simulink model "Filter_attivo"  (R2016b)
settings: Solver=ode23t  StartTime=0.0  StopTime=2.4  MaxStep=1e-4  RelTol=1e-3  EnableMultiTasking=on
values from neighbouring files (symbols this model uses):
  ampiezza_rete = 150/sqrt(3)    [Data.m]    (also in taratura.m)
  C = 2.2e-3    (= 0.0022)    [Data.m]
  C_raddr = 600e-6    (= 0.0006)    [Data.m]
  f = 50    [Data.m]    (also in Spettro_complesso.m = bar(-fp((26:25:25000-25)),PyTHD(length(PyTHD)-1:-1:length(Py)
  f_am = 500    [Data.m]
  h = Lagrange_coef(f,1/Tc)    [Data.m]    (also in Lagrange_coef.m = NaN(4,round(fc/f1*0.5)))
  h_rit = Lagrange_coef_rit(1.5)    [Data.m]
  k_interno = 0.99    [tuning.m]
  k_par_AM = 10    [Data.m]
  ki_PI = 0.2    [Data.m]
  ki_PLL = 1000    [Data.m]
  ki_ris = 47.5*2    (= 95)    [Data.m]
  kp_PI = 1.57    [Data.m]
  kp_PLL = 0.9    [Data.m]
  kp_ris = 47.5*0.089*2    (= 8.455)    [Data.m]
  L_disaccoppiamento = 2*1.18e-3    (= 0.00236)    [Data.m]    (also in taratura.m)
  L_rete = 4e-3    (= 0.004)    [Data.m]    (also in tuning.m)
  max_PI = 8    [Data.m]
  max_PLL = 1000    [Data.m]
  min_PI = -8    [Data.m]
  min_PLL = -1000    [Data.m]
  Notch_z = 1-Peaking_z    [Data.m]
  Notch_z_AM1 = 1-Peaking_z_AM1    [Notch.m]
  peak_rete = Peaking(f,1/Tc,0.1)    [Data.m]
  Peaking_dir1_d = c2d(Peaking_dir1_s,1/fs,'tustin')    [semipeaking.m]
  pendenza = 1000    [Data.m]
  R_carico = 50    [Data.m]
  R_disaccoppiamento = 2*13e-3    (= 0.026)    [Data.m]    (also in taratura.m)
  R_raddr = 60    [Data.m]
  R_rete = 100e-3    (= 0.1)    [Data.m]    (also in tuning.m = 0.01)
  T = 20e-3    (= 0.02)    [Data.m]    (also in tuning.m)
  tau_filtro_Vdc_ref = 0.15    [Data.m]
  Tc = 1/10000    (= 0.0001)    [Data.m]    (also in taratura.m; tuning.m)
  Vdc_ref = 200    [Data.m]    (also in taratura.m)
  w_filtro = 2*pi*f_taglio    (= 56548.6677646)    [Data.m]
undefined symbols (not defined in the file or in its folder): DiscIntNeverNeededParam, k_par, k_ser, Notch_z_AM1_5, Notch_z_AM1_7, Notch_z_AM2_5, Notch_z_AM2_7, Peaking_inv_d, plecs, Q_inv
libraries: powerlib x54, simulink x8, powerlib_extras x4, powerlib_meascontrol x2
(part 1 of 5)
settings Model: SimulationMode=accelerator  Creator=utente  LastModifiedBy=franc
settings DataIOCC: SaveFormat=Array
settings OptimizationCC: ExpressionDepthLimit=2147483647  EfficientMapNaN2IntZero=off  LifeSpan=inf
settings DebuggingCC: UnderspecifiedInitializationDetection=Classic  MergeDetectMultiDrivingBlocksExec=none  MaxConsecutiveZCsMsg=none  SolverPrmCheckMsg=warning  FcnCallInpInsideContextMsg=warning  AllowSymbolicDim=off  StateNameClashWarn=warning  SFUnexpectedBacktrackingDiag=warning  SFNoUnconditionalDefaultTransitionDiag=warning  SFExecutionAtInitializationDiag=none
settings HardwareCC: ProdBitPerPointer=32  ProdBitPerSizeT=32  ProdBitPerPtrDiffT=32  ProdLargestAtomicFloat=None  ProdIntDivRoundTo=Undefined  ProdEndianess=Unspecified  ProdWordSize=32  ProdHWDeviceType=32-bit Generic  TargetBitPerPointer=64  TargetBitPerSizeT=64  TargetBitPerPtrDiffT=64  TargetLongLongMode=on  TargetIntDivRoundTo=Zero  TargetEndianess=LittleEndian  TargetWordSize=64  TargetHWDeviceType=MATLAB Host  ProdEqTarget=off
settings ModelReferenceCC: PropagateSignalLabelsOutOfModel=off
settings SFSimCC: SimParseCustomCode=off
settings CodeAppCC: MaxIdLength=128
settings GRTTargetCC: TargetLangStandard=C89/C90 (ANSI)  CombineOutputUpdateFcns=off  GRTInterface=on
settings ConfigComp: CovMetricSettings=dw  CovHtmlReporting=on  CovSaveCumulativeToWorkspaceVar=on  CovSaveSingleToWorkspaceVar=on  CovExternalEMLEnable=off  CovSFcnEnable=off

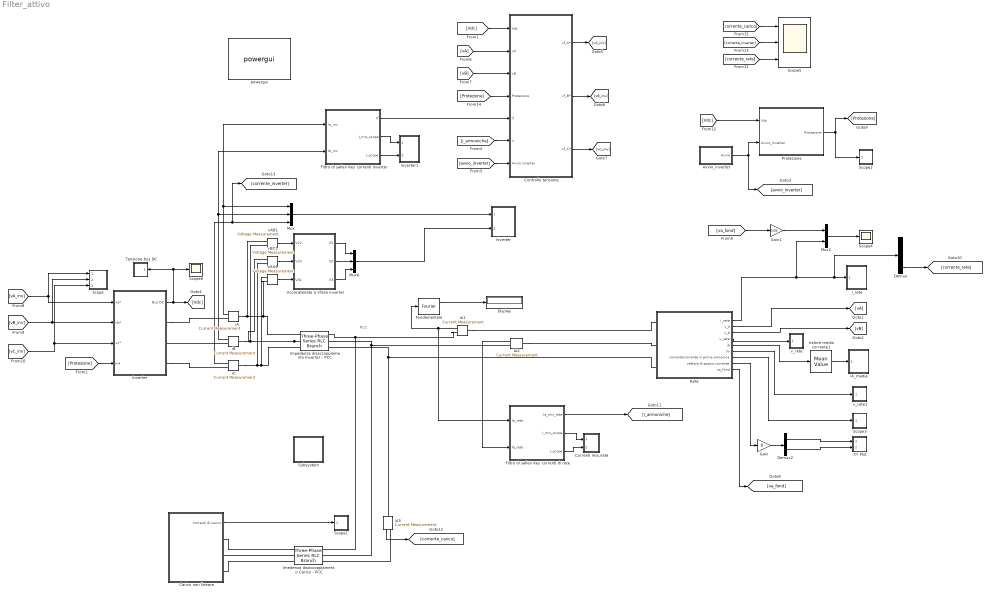
== system Filter_attivo ==
  note: PCC
  Avvio_inverter : Subsystem  mask{avvio=0.2}
      mask prompts: avvio "Istante avvio inverter"
  Carico non lineare : Subsystem
  Controllo tensione : Subsystem
  Correnti misurate : Subsystem  LoadFcn=plecs('sl', 300);  InitFcn=plecs('sl', 314);  StartFcn=plecs('sl', 308);  StopFcn=plecs('sl', 309);  mask{Settings=<binary blob, 300 chars, not shown>}
      mask init:
      | plecs('sl', 315);
      settings: CopyFcn=plecs('sl', 303);  DeleteFcn=plecs('sl', 305);  UndoDeleteFcn=plecs('sl', 306);  PreSaveFcn=plecs('sl', 311);  NameChangeFcn=plecs('sl', 310);  DestroyFcn=plecs('sl', 307);  OpenFcn=plecs('sl', 302);  ErrorFcn=plerrorfcn
      mask Display: plot([0.1 0.9 0.9 0.1 0.1], [0.9 0.9 0.5 0.5 0.9])
  Demux : Demux  Outputs=3
  Demux2 : Demux  Outputs=2
  Display : Display
  "Filtro di sallen Key correnti inverter " : Subsystem
  Filtro di sallen Key correnti di rete : Subsystem
  Fondamentale : powerlib_meascontrol/Measurements/Fourier  Freq=50  n=1  InInit=[0, 0]  Ts=0
  Gain : Gain  Gain=0
  Gain1 : Gain  Gain=0.05
  Imedenza disaccoppiamento Carico - PCC : powerlib/Elements/Three-Phase Series RLC Branch  LConnTagsString=A|B|C  RConnTagsString=A|B|C  BranchType=RL  Resistance=R_disaccoppiamento  Inductance=L_disaccoppiamento  Capacitance=1e-6  Measurements=None
  Impedenza disaccoppiamento Inverter - PCC : powerlib/Elements/Three-Phase Series RLC Branch  LConnTagsString=A|B|C  RConnTagsString=A|B|C  BranchType=RL  Resistance=R_disaccoppiamento  Inductance=L_disaccoppiamento  Capacitance=1e-6  Measurements=None
  Inverter : Subsystem  LoadFcn=plecs('sl', 300);  InitFcn=plecs('sl', 314);  StartFcn=plecs('sl', 308);  StopFcn=plecs('sl', 309);  mask{Settings=<binary blob, 1152 chars, not shown>}
      mask init:
      | plecs('sl', 315);
      settings: CopyFcn=plecs('sl', 303);  DeleteFcn=plecs('sl', 305);  UndoDeleteFcn=plecs('sl', 306);  PreSaveFcn=plecs('sl', 311);  NameChangeFcn=plecs('sl', 310);  DestroyFcn=plecs('sl', 307);  OpenFcn=plecs('sl', 302);  ErrorFcn=plerrorfcn
      mask Display: plot([0.1 0.9 0.9 0.1 0.1], [0.9 0.9 0.5 0.5 0.9])
  "Inverter " : Subsystem
  Inverter1 : Subsystem  LoadFcn=plecs('sl', 300);  InitFcn=plecs('sl', 314);  StartFcn=plecs('sl', 308);  StopFcn=plecs('sl', 309);  mask{Settings=<binary blob, 1020 chars, not shown>}
      mask init:
      | plecs('sl', 315);
      settings: CopyFcn=plecs('sl', 303);  DeleteFcn=plecs('sl', 305);  UndoDeleteFcn=plecs('sl', 306);  PreSaveFcn=plecs('sl', 311);  NameChangeFcn=plecs('sl', 310);  DestroyFcn=plecs('sl', 307);  OpenFcn=plecs('sl', 302);  ErrorFcn=plerrorfcn
      mask Display: plot([0.1 0.9 0.9 0.1 0.1], [0.9 0.9 0.5 0.5 0.9])
  Mux : Mux  Inputs=3
  Mux2 : Mux  Inputs=2
  Mux6 : Mux  Inputs=3
  Protezione : Subsystem  mask{limite_up=250, limite_down=70}
      mask prompts: limite_up "tensione max bus DC"; limite_down "tensione min bus DC"
  Rete : Subsystem
  Scope : Subsystem  LoadFcn=plecs('sl', 300);  InitFcn=plecs('sl', 314);  StartFcn=plecs('sl', 308);  StopFcn=plecs('sl', 309);  mask{Settings=<binary blob, 1148 chars, not shown>}
      mask init:
      | plecs('sl', 315);
      settings: CopyFcn=plecs('sl', 303);  DeleteFcn=plecs('sl', 305);  UndoDeleteFcn=plecs('sl', 306);  PreSaveFcn=plecs('sl', 311);  NameChangeFcn=plecs('sl', 310);  DestroyFcn=plecs('sl', 307);  OpenFcn=plecs('sl', 302);  ErrorFcn=plerrorfcn
      mask Display: plot([0.1 0.9 0.9 0.1 0.1], [0.9 0.9 0.5 0.5 0.9])
  Scope1 : Subsystem  LoadFcn=plecs('sl', 300);  InitFcn=plecs('sl', 314);  StartFcn=plecs('sl', 308);  StopFcn=plecs('sl', 309);  mask{Settings=<binary blob, 876 chars, not shown>}
      mask init:
      | plecs('sl', 315);
      settings: CopyFcn=plecs('sl', 303);  DeleteFcn=plecs('sl', 305);  UndoDeleteFcn=plecs('sl', 306);  PreSaveFcn=plecs('sl', 311);  NameChangeFcn=plecs('sl', 310);  DestroyFcn=plecs('sl', 307);  OpenFcn=plecs('sl', 302);  ErrorFcn=plerrorfcn
      mask Display: plot([0.1 0.9 0.9 0.1 0.1], [0.9 0.9 0.5 0.5 0.9])
  Scope2 : Subsystem  LoadFcn=plecs('sl', 300);  InitFcn=plecs('sl', 314);  StartFcn=plecs('sl', 308);  StopFcn=plecs('sl', 309);  mask{Settings=<binary blob, 892 chars, not shown>}
      mask init:
      | plecs('sl', 315);
      settings: CopyFcn=plecs('sl', 303);  DeleteFcn=plecs('sl', 305);  UndoDeleteFcn=plecs('sl', 306);  PreSaveFcn=plecs('sl', 311);  NameChangeFcn=plecs('sl', 310);  DestroyFcn=plecs('sl', 307);  OpenFcn=plecs('sl', 302);  ErrorFcn=plerrorfcn
      mask Display: plot([0.1 0.9 0.9 0.1 0.1], [0.9 0.9 0.5 0.5 0.9])
  Scope3 : Subsystem  LoadFcn=plecs('sl', 300);  InitFcn=plecs('sl', 314);  StartFcn=plecs('sl', 308);  StopFcn=plecs('sl', 309);  mask{Settings=<binary blob, 892 chars, not shown>}
      mask init:
      | plecs('sl', 315);
      settings: CopyFcn=plecs('sl', 303);  DeleteFcn=plecs('sl', 305);  UndoDeleteFcn=plecs('sl', 306);  PreSaveFcn=plecs('sl', 311);  NameChangeFcn=plecs('sl', 310);  DestroyFcn=plecs('sl', 307);  OpenFcn=plecs('sl', 302);  ErrorFcn=plerrorfcn
      mask Display: plot([0.1 0.9 0.9 0.1 0.1], [0.9 0.9 0.5 0.5 0.9])
  Scope4 : Scope
  Scope5 : Scope  NumInputPorts=3
  Scope6 : Scope
  Subsystem : Subsystem
  Tensione bus DC : Subsystem  LoadFcn=plecs('sl', 300);  InitFcn=plecs('sl', 314);  StartFcn=plecs('sl', 308);  StopFcn=plecs('sl', 309);  mask{Settings=<binary blob, 960 chars, not shown>}
      mask init:
      | plecs('sl', 315);
      settings: CopyFcn=plecs('sl', 303);  DeleteFcn=plecs('sl', 305);  UndoDeleteFcn=plecs('sl', 306);  PreSaveFcn=plecs('sl', 311);  NameChangeFcn=plecs('sl', 310);  DestroyFcn=plecs('sl', 307);  OpenFcn=plecs('sl', 302);  ErrorFcn=plerrorfcn
      mask Display: plot([0.1 0.9 0.9 0.1 0.1], [0.9 0.9 0.5 0.5 0.9])
  Valore medio corrente1 : powerlib_extras/Measurements/Mean Value  Period=3*Tc
  Vconcatenate a Vfase inverter : Subsystem
  XY Plot : Subsystem  LoadFcn=plecs('sl', 317);  InitFcn=plecs('sl', 314);  StartFcn=plecs('sl', 308);  StopFcn=plecs('sl', 309);  mask{Settings=<binary blob, 592 chars, not shown>}
      mask init:
      | plecs('sl', 315);
      settings: CopyFcn=plecs('sl', 318);  DeleteFcn=plecs('sl', 305);  UndoDeleteFcn=plecs('sl', 306);  PreSaveFcn=plecs('sl', 311);  NameChangeFcn=plecs('sl', 310);  DestroyFcn=plecs('sl', 307);  OpenFcn=plecs('sl', 302);  ErrorFcn=plerrorfcn
      mask Display:
      | plot([0.05 0.95 0.95 0.05 0.05], [0.95 0.95 0.05 0.05 0.95])
      | plot(0.5+sin((0:0.2:2)*pi)*0.3, 0.5+sin((0:0.2:2)*pi + pi/4)*0.3);
  iA{,1..2,5} (4 alike) : powerlib/Measurements/Current Measurement  PhasorSimulation=off  OutputType=Complex  PSBequivalent=0
  iA_media : Subsystem  LoadFcn=plecs('sl', 300);  InitFcn=plecs('sl', 314);  StartFcn=plecs('sl', 308);  StopFcn=plecs('sl', 309);  mask{Settings=<binary blob, 892 chars, not shown>}
      mask init:
      | plecs('sl', 315);
      settings: CopyFcn=plecs('sl', 303);  DeleteFcn=plecs('sl', 305);  UndoDeleteFcn=plecs('sl', 306);  PreSaveFcn=plecs('sl', 311);  NameChangeFcn=plecs('sl', 310);  DestroyFcn=plecs('sl', 307);  OpenFcn=plecs('sl', 302);  ErrorFcn=plerrorfcn
      mask Display: plot([0.1 0.9 0.9 0.1 0.1], [0.9 0.9 0.5 0.5 0.9])
  iB : powerlib/Measurements/Current Measurement  PhasorSimulation=off  OutputType=Complex  PSBequivalent=0
  iC : powerlib/Measurements/Current Measurement  PhasorSimulation=off  OutputType=Complex  PSBequivalent=0
  i_rete : Subsystem  LoadFcn=plecs('sl', 300);  InitFcn=plecs('sl', 314);  StartFcn=plecs('sl', 308);  StopFcn=plecs('sl', 309);  mask{Settings=<binary blob, 1020 chars, not shown>}
      mask init:
      | plecs('sl', 315);
      settings: CopyFcn=plecs('sl', 303);  DeleteFcn=plecs('sl', 305);  UndoDeleteFcn=plecs('sl', 306);  PreSaveFcn=plecs('sl', 311);  NameChangeFcn=plecs('sl', 310);  DestroyFcn=plecs('sl', 307);  OpenFcn=plecs('sl', 302);  ErrorFcn=plerrorfcn
      mask Display: plot([0.1 0.9 0.9 0.1 0.1], [0.9 0.9 0.5 0.5 0.9])
  powergui : powerlib/powergui  SimulationMode=Continuous  SolverType=Tustin  SampleTime=50e-6  frequency=60  SPID=off  DisableSnubberDevices=off  DisableRonSwitches=off  DisableVfSwitches=off  SwTol=0  DisplayEquations=off  Interpol=off  ExternalGateDelay=off  methode=off  Ts=0  FunctionMessages=off  echomessages=off  HookPort=off  EnableUseOfTLC=off  x0status=blocks  frequencyindice=0  Pbase=100e6  ErrMax=1e-4  Iterations=50  UnitsV=kV  UnitsW=MW  buscounter=0  RestoreLinks=warning  ResistiveCurrentMeasurement=off  Frange=[0:2:500]  Ylog=off  Xlog=on  ShowGrid=off  save=off  variable=ZData  structure=logsout  ZoomFFT=off  StartTime=1  cycles=5  DisplayStyle=1  fundamental=50  FreqAxis=off  MaxFrequency=10000  frequencyindicesteady=1  RmsSteady=1  display=off
  vAB1 : powerlib/Measurements/Voltage Measurement  PhasorSimulation=off  OutputType=Complex  PSBequivalent=0
  vBC1 : powerlib/Measurements/Voltage Measurement  PhasorSimulation=off  OutputType=Complex  PSBequivalent=0
  vCA1 : powerlib/Measurements/Voltage Measurement  PhasorSimulation=off  OutputType=Complex  PSBequivalent=0
  v_rete : Subsystem  LoadFcn=plecs('sl', 300);  InitFcn=plecs('sl', 314);  StartFcn=plecs('sl', 308);  StopFcn=plecs('sl', 309);  mask{Settings=<binary blob, 892 chars, not shown>}
      mask init:
      | plecs('sl', 315);
      settings: CopyFcn=plecs('sl', 303);  DeleteFcn=plecs('sl', 305);  UndoDeleteFcn=plecs('sl', 306);  PreSaveFcn=plecs('sl', 311);  NameChangeFcn=plecs('sl', 310);  DestroyFcn=plecs('sl', 307);  OpenFcn=plecs('sl', 302);  ErrorFcn=plerrorfcn
      mask Display: plot([0.1 0.9 0.9 0.1 0.1], [0.9 0.9 0.5 0.5 0.9])
  v_rete1 : Subsystem  LoadFcn=plecs('sl', 300);  InitFcn=plecs('sl', 314);  StartFcn=plecs('sl', 308);  StopFcn=plecs('sl', 309);  mask{Settings=<binary blob, 892 chars, not shown>}
      mask init:
      | plecs('sl', 315);
      settings: CopyFcn=plecs('sl', 303);  DeleteFcn=plecs('sl', 305);  UndoDeleteFcn=plecs('sl', 306);  PreSaveFcn=plecs('sl', 311);  NameChangeFcn=plecs('sl', 310);  DestroyFcn=plecs('sl', 307);  OpenFcn=plecs('sl', 302);  ErrorFcn=plerrorfcn
      mask Display: plot([0.1 0.9 0.9 0.1 0.1], [0.9 0.9 0.5 0.5 0.9])
  wires:
  [Vdc] -> Controllo tensione/1(Vdc)
  iB/1 -> "Filtro di sallen Key correnti inverter "/2(Ib_inv), Mux/2
  iA/1 -> "Filtro di sallen Key correnti inverter "/1(Ia_inv), Mux/1
  [vA] -> Controllo tensione/2(vA)
  [vB] -> Controllo tensione/3(vB)
  iC/1 -> [corrente_inverter], Mux/3
  Controllo tensione/3(vf_C*) -> [vC_inv]
  Controllo tensione/2(vf_B*) -> [vB_inv]
  Controllo tensione/1(vf_A*) -> [vA_inv]
  [Protezione] -> Controllo tensione/4(Protezione)
  vAB1/1 -> Vconcatenate a Vfase inverter/1(V12)
  vBC1/1 -> Vconcatenate a Vfase inverter/2(V23)
  vCA1/1 -> Vconcatenate a Vfase inverter/3(V31)
  Vconcatenate a Vfase inverter/2(E2) -> Mux6/2
  Vconcatenate a Vfase inverter/1(E1) -> Mux6/1
  Vconcatenate a Vfase inverter/3(E3) -> Mux6/3
  "Filtro di sallen Key correnti inverter "/2(I_mis_scope) -> Inverter1/1(1)
  "Filtro di sallen Key correnti inverter "/3(I_scope) -> Inverter1/2(2)
  "Filtro di sallen Key correnti inverter "/1(If) -> Controllo tensione/5(if)
  Protezione/1("Protezione ") -> Scope2/1(1), [Protezione]
  [Vdc] -> Protezione/1(Vdc)
  [vA_inv] -> Scope/1(1), "Inverter "/1(va*)
  [vB_inv] -> Scope/2(2), "Inverter "/2(vb*)
  [vC_inv] -> Scope/3(3), "Inverter "/3(vc*)
  [Protezione] -> "Inverter "/4(In4)
  "Inverter "/1(Bus DC) -> Scope6/1, Tensione bus DC/1(1), [Vdc]
  Rete/2(v_a) -> [vA]
  Rete/3(v_b) -> [vB]
  [i_armoniche] -> Controllo tensione/6(ir)
  iA1/1 -> Filtro di sallen Key correnti di rete/1(Ia_rete), Fondamentale/1
  Carico non lineare/1(Correnti di carico) -> Scope1/1(1)
  Fondamentale/1 -> Display/1
  iA2/1 -> Filtro di sallen Key correnti di rete/2(Ib_rete)
  Filtro di sallen Key correnti di rete/2(I_mis_scope) -> Correnti misurate/1(1)
  Filtro di sallen Key correnti di rete/3(I_scope) -> Correnti misurate/2(2)
  Filtro di sallen Key correnti di rete/1(Ia_mis_rete) -> [i_armoniche]
  Rete/4("v_rete ") -> v_rete/1(1)
  iA5/1 -> [corrente_carico]
  Rete/1("i_rete ") -> Mux2/2, Demux/1, i_rete/1(1)
  Avvio_inverter/1(Avvio) -> [avvio_inverter], Protezione/2(Avvio_inverter)
  Mux/1 -> Inverter/1(1)
  Mux6/1 -> Inverter/2(2)
  Rete/5(iA) -> Valore medio corrente1/1
  Valore medio corrente1/1 -> iA_media/1(1)
  [avvio_inverter] -> Controllo tensione/7("Avvio inverter ")
  Rete/6(i/v) -> v_rete1/1(1)
  Rete/7(corrente/corrente in prima armonica) -> Scope3/1(1)
  Rete/8(vettore di spazio corrente) -> Gain/1
  Demux2/1 -> XY Plot/1(1)
  Demux2/2 -> XY Plot/2(2)
  Gain/1 -> Demux2/1
  Mux2/1 -> Scope4/1
  Gain1/1 -> Mux2/1
  [va_fond] -> Gain1/1
  Rete/9(va_fond) -> [va_fond]
  Demux/3 -> [corrente_rete]
  [corrente_rete] -> Scope5/3
  [corrente_inverter] -> Scope5/2
  [corrente_carico] -> Scope5/1
  connections:
  vAB1/LConn1 -- iA/LConn1 -- vCA1/LConn2 -- Impedenza disaccoppiamento Inverter - PCC/LConn1
  Impedenza disaccoppiamento Inverter - PCC/LConn2 -- iB/LConn1 -- vBC1/LConn1 -- vAB1/LConn2
  vBC1/LConn2 -- vCA1/LConn1 -- Impedenza disaccoppiamento Inverter - PCC/LConn3 -- iC/LConn1
  Imedenza disaccoppiamento Carico - PCC/LConn2 -- Carico non lineare/RConn2
  Carico non lineare/RConn1 -- Imedenza disaccoppiamento Carico - PCC/LConn1
  Carico non lineare/RConn3 -- Imedenza disaccoppiamento Carico - PCC/LConn3
  iA2/LConn1 -- Rete/LConn2
  Rete/LConn3 -- iA5/LConn1 -- Impedenza disaccoppiamento Inverter - PCC/RConn3
  iA1/LConn1 -- Rete/LConn1
  iA1/RConn1 -- Imedenza disaccoppiamento Carico - PCC/RConn1 -- Impedenza disaccoppiamento Inverter - PCC/RConn1
  Impedenza disaccoppiamento Inverter - PCC/RConn2 -- Imedenza disaccoppiamento Carico - PCC/RConn2 -- iA2/RConn1
  iA5/RConn1 -- Imedenza disaccoppiamento Carico - PCC/RConn3
  "Inverter "/RConn1 -- iA/RConn1
  iB/RConn1 -- "Inverter "/RConn2
  "Inverter "/RConn3 -- iC/RConn1

== system Filter_attivo/Avvio_inverter ==
  Compare To Constant : simulink/Logic and Bit Operations/Compare To Constant  relop=>  const=avvio  OutDataTypeStr=uint8  ZeroCross=off
  Constant1 : Constant
  Integrator : Integrator  LimitOutput=on  UpperSaturationLimit=20  LowerSaturationLimit=-20
  Avvio : Outport
  wires:
  Constant1/1 -> Integrator/1
  Integrator/1 -> Compare To Constant/1
  Compare To Constant/1 -> Avvio/1

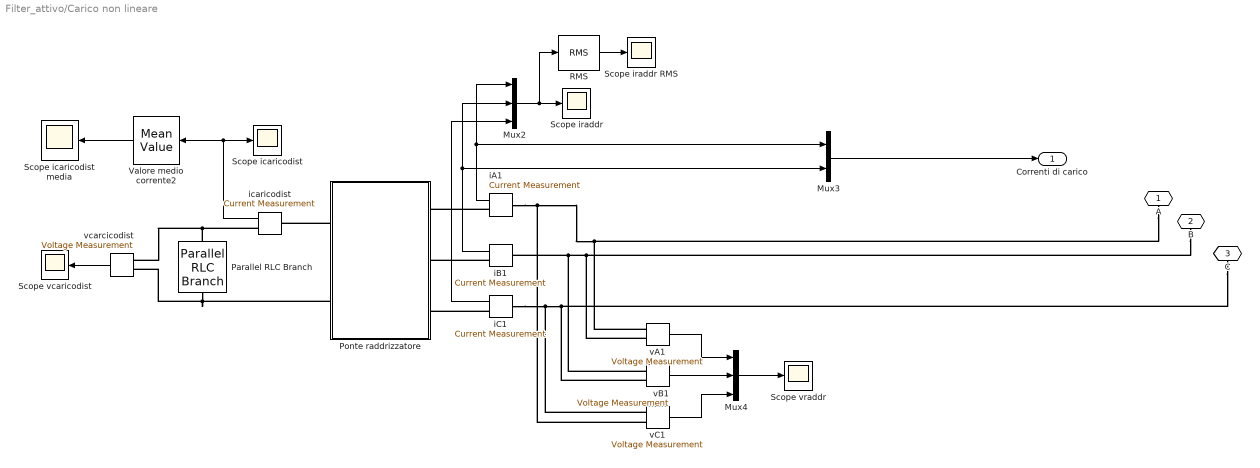
== system Filter_attivo/Carico non lineare ==
  Mux2 : Mux  Inputs=3
  Mux3 : Mux  Inputs=2
  Mux4 : Mux  Inputs=3
  Parallel RLC Branch : powerlib/Elements/Parallel RLC Branch  LConnTagsString=a  RConnTagsString=__new0  BranchType=RC  Resistance=R_raddr  Inductance=1e-3  SetiL0=off  InitialCurrent=0  Capacitance=C_raddr  Setx0=on  InitialVoltage=V_cond_iniz  Measurements=None
  Ponte raddrizzatore : Subsystem
  RMS : powerlib_extras/Measurements/RMS  f1=50
  Scope icaricodist : Scope
  Scope icaricodist media : Scope
  Scope vcaricodist : Scope
  Scope iraddr : Scope
  Scope iraddr RMS : Scope
  Scope vraddr : Scope
  Valore medio corrente2 : powerlib_extras/Measurements/Mean Value  Period=3*Tc
  iA1 : powerlib/Measurements/Current Measurement  PhasorSimulation=off  OutputType=Complex  PSBequivalent=0
  iB1 : powerlib/Measurements/Current Measurement  PhasorSimulation=off  OutputType=Complex  PSBequivalent=0
  iC1 : powerlib/Measurements/Current Measurement  PhasorSimulation=off  OutputType=Complex  PSBequivalent=0
  icaricodist : powerlib/Measurements/Current Measurement  PhasorSimulation=off  OutputType=Complex  PSBequivalent=0
  vA1 : powerlib/Measurements/Voltage Measurement  PhasorSimulation=off  OutputType=Complex  PSBequivalent=0
  vB1 : powerlib/Measurements/Voltage Measurement  PhasorSimulation=off  OutputType=Complex  PSBequivalent=0
  vC1 : powerlib/Measurements/Voltage Measurement  PhasorSimulation=off  OutputType=Complex  PSBequivalent=0
  vcarcicodist : powerlib/Measurements/Voltage Measurement  PhasorSimulation=off  OutputType=Complex  PSBequivalent=0
  A : PMIOPort  Port=1  Side=Right
  B : PMIOPort  Port=2  Side=Right
  C : PMIOPort  Port=3  Side=Right
  Correnti di carico : Outport
  wires:
  iC1/1 -> Mux2/3
  Mux2/1 -> Scope iraddr/1, RMS/1
  vcarcicodist/1 -> Scope vcaricodist/1
  RMS/1 -> Scope iraddr RMS/1
  vB1/1 -> Mux4/2
  vA1/1 -> Mux4/1
  vC1/1 -> Mux4/3
  Mux4/1 -> Scope vraddr/1
  Valore medio corrente2/1 -> Scope icaricodist media/1
  icaricodist/1 -> Scope icaricodist/1, Valore medio corrente2/1
  iA1/1 -> Mux2/1, Mux3/1
  iB1/1 -> Mux2/2, Mux3/2
  Mux3/1 -> Correnti di carico/1
  connections:
  iA1/LConn1 -- A/RConn1 -- vA1/LConn1 -- vC1/LConn2
  iB1/RConn1 -- Ponte raddrizzatore/LConn2
  icaricodist/RConn1 -- Parallel RLC Branch/RConn1 -- vcarcicodist/LConn1
  vA1/LConn2 -- B/RConn1 -- vB1/LConn1 -- iB1/LConn1
  iA1/RConn1 -- Ponte raddrizzatore/LConn1
  iC1/RConn1 -- Ponte raddrizzatore/LConn3
  iC1/LConn1 -- C/RConn1 -- vB1/LConn2 -- vC1/LConn1
  Ponte raddrizzatore/RConn2 -- Parallel RLC Branch/LConn1 -- vcarcicodist/LConn2
  Ponte raddrizzatore/RConn1 -- icaricodist/LConn1

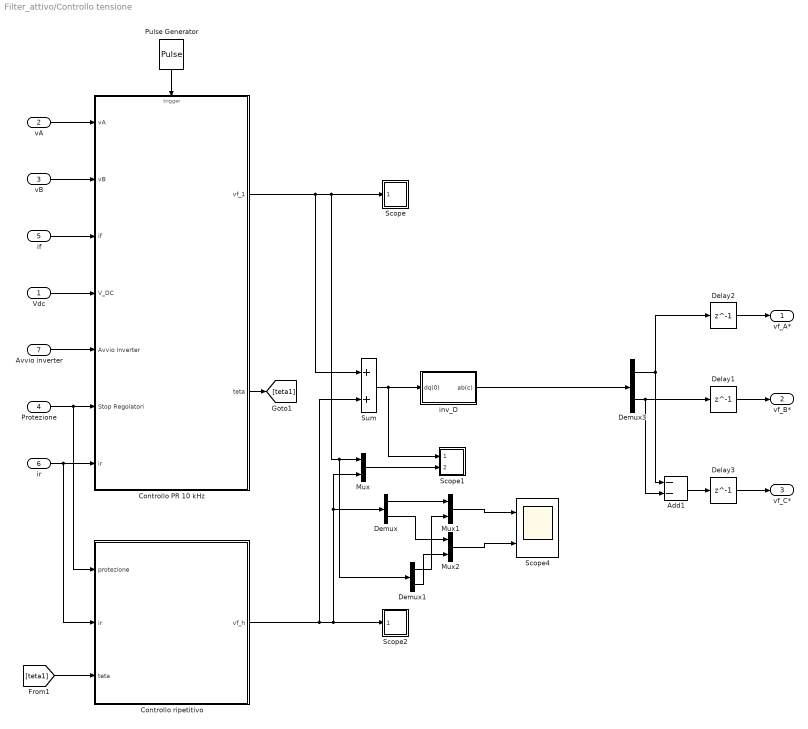
== system Filter_attivo/Controllo tensione ==
  Vdc : Inport
  vA : Inport  Port=2
  vB : Inport  Port=3
  Protezione : Inport  Port=4
  if : Inport  Port=5
  ir : Inport  Port=6
  "Avvio inverter " : Inport  Port=7
  Add1 : Sum  Inputs=--
  Controllo PR 10 kHz : Subsystem
  Controllo ripetitivo : Subsystem  mask{down=3, time_to_rip=0.4, k_serie_d=5, alfa=0}
      mask prompts: down "Ordine del Downsapling"; time_to_rip "Avvio ripetitivo"; k_serie_d "k_serie"; alfa "0 per controllo normale, 1 per downsampling"
  Delay1 : Delay  DelayLength=1
  Delay2 : Delay  DelayLength=1
  Delay3 : Delay  DelayLength=1
  Demux : Demux  Outputs=2
  Demux1 : Demux  Outputs=2
  Demux3 : Demux  Outputs=2
  Mux : Mux  Inputs=2
  Mux1 : Mux  Inputs=2
  Mux2 : Mux  Inputs=2
  Pulse Generator : DiscretePulseGenerator  PulseType=Time based  Period=Tc
  Scope : Subsystem  LoadFcn=plecs('sl', 300);  InitFcn=plecs('sl', 314);  StartFcn=plecs('sl', 308);  StopFcn=plecs('sl', 309);  mask{Settings=<binary blob, 892 chars, not shown>}
      mask init:
      | plecs('sl', 315);
      settings: CopyFcn=plecs('sl', 303);  DeleteFcn=plecs('sl', 305);  UndoDeleteFcn=plecs('sl', 306);  PreSaveFcn=plecs('sl', 311);  NameChangeFcn=plecs('sl', 310);  DestroyFcn=plecs('sl', 307);  OpenFcn=plecs('sl', 302);  ErrorFcn=plerrorfcn
      mask Display: plot([0.1 0.9 0.9 0.1 0.1], [0.9 0.9 0.5 0.5 0.9])
  Scope1 : Subsystem  LoadFcn=plecs('sl', 300);  InitFcn=plecs('sl', 314);  StartFcn=plecs('sl', 308);  StopFcn=plecs('sl', 309);  mask{Settings=<binary blob, 1152 chars, not shown>}
      mask init:
      | plecs('sl', 315);
      settings: CopyFcn=plecs('sl', 303);  DeleteFcn=plecs('sl', 305);  UndoDeleteFcn=plecs('sl', 306);  PreSaveFcn=plecs('sl', 311);  NameChangeFcn=plecs('sl', 310);  DestroyFcn=plecs('sl', 307);  OpenFcn=plecs('sl', 302);  ErrorFcn=plerrorfcn
      mask Display: plot([0.1 0.9 0.9 0.1 0.1], [0.9 0.9 0.5 0.5 0.9])
  Scope2 : Subsystem  LoadFcn=plecs('sl', 300);  InitFcn=plecs('sl', 314);  StartFcn=plecs('sl', 308);  StopFcn=plecs('sl', 309);  mask{Settings=<binary blob, 892 chars, not shown>}
      mask init:
      | plecs('sl', 315);
      settings: CopyFcn=plecs('sl', 303);  DeleteFcn=plecs('sl', 305);  UndoDeleteFcn=plecs('sl', 306);  PreSaveFcn=plecs('sl', 311);  NameChangeFcn=plecs('sl', 310);  DestroyFcn=plecs('sl', 307);  OpenFcn=plecs('sl', 302);  ErrorFcn=plerrorfcn
      mask Display: plot([0.1 0.9 0.9 0.1 0.1], [0.9 0.9 0.5 0.5 0.9])
  Scope4 : Scope  NumInputPorts=2
  Sum : Sum
  inv_D : Subsystem
  vf_A* : Outport
  vf_B* : Outport  Port=2
  vf_C* : Outport  Port=3
  wires:
  Delay2/1 -> vf_A*/1
  Delay1/1 -> vf_B*/1
  Delay3/1 -> vf_C*/1
  Pulse Generator/1 -> Controllo PR 10 kHz/Trigger
  vA/1 -> Controllo PR 10 kHz/1(vA)
  vB/1 -> Controllo PR 10 kHz/2(vB)
  if/1 -> Controllo PR 10 kHz/3(if)
  Vdc/1 -> Controllo PR 10 kHz/4(V_DC)
  "Avvio inverter "/1 -> Controllo PR 10 kHz/5(Avvio Inverter)
  ir/1 -> Controllo ripetitivo/2(ir), Controllo PR 10 kHz/7(ir)
  Protezione/1 -> Controllo PR 10 kHz/6(Stop Regolatori), Controllo ripetitivo/1(protezione)
  Demux3/1 -> Delay2/1, Add1/1
  Demux3/2 -> Delay1/1, Add1/2
  Add1/1 -> Delay3/1
  inv_D/1(ab(c)) -> Demux3/1
  Controllo PR 10 kHz/1(vf_1) -> Demux1/1, Mux/1, Scope/1(1), Sum/1
  Sum/1 -> Scope1/1(1), inv_D/1(dq(0))
  Controllo PR 10 kHz/2(teta) -> [teta1]
  Controllo ripetitivo/1(vf_h) -> Demux/1, Mux/2, Scope2/1(1), Sum/2
  [teta1] -> Controllo ripetitivo/3(teta)
  Mux/1 -> Scope1/2(2)
  Demux/1 -> Mux1/1
  Demux1/1 -> Mux1/2
  Demux/2 -> Mux2/1
  Demux1/2 -> Mux2/2
  Mux1/1 -> Scope4/1
  Mux2/1 -> Scope4/2

== system Filter_attivo/Correnti misurate ==
  1 : Inport
  2 : Inport  Port=2
  " 1 " : DataTypeConversion  SaturateOnIntegerOverflow=on  RndMeth=Zero
  " 2 " : DataTypeConversion  SaturateOnIntegerOverflow=on  RndMeth=Zero
  " InputMux " : Mux  Inputs=2
  " S-Function " : S-Function  FunctionName=plecs  SFunctionDeploymentMode=off  EnableBusSupport=off
  wires:
  " 2 "/1 -> " InputMux "/2
  2/1 -> " 2 "/1
  " 1 "/1 -> " InputMux "/1
  1/1 -> " 1 "/1
  " InputMux "/1 -> " S-Function "/1

== system Filter_attivo/Filtro di sallen Key correnti inverter  ==
  Ia_inv : Inport
  Ib_inv : Inport  Port=2
  D : Subsystem
  Fase_A : TransferFcn  Denominator=[1/(w_filtro)^2 2/w_filtro 1]
  Fase_B : TransferFcn  Denominator=[1/(w_filtro)^2 2/w_filtro 1]
  Mux1 : Mux  Inputs=2
  Mux14 : Mux  Inputs=2
  Mux2 : Mux  Inputs=2
  If : Outport
  I_mis_scope : Outport  Port=2
  I_scope : Outport  Port=3
  wires:
  Ib_inv/1 -> Mux2/2, Fase_B/1
  Fase_A/1 -> Mux1/1, Mux14/1
  Mux14/1 -> I_mis_scope/1
  Mux2/1 -> I_scope/1
  Ia_inv/1 -> Fase_A/1, Mux2/1
  Fase_B/1 -> Mux1/2, Mux14/2
  Mux1/1 -> D/1(ab(c))
  D/1(dq(0)) -> If/1

== system Filter_attivo/Filtro di sallen Key correnti di rete ==
  Ia_rete : Inport
  Ib_rete : Inport  Port=2
  Fase_A : TransferFcn  Denominator=[1/(w_filtro)^2 2/w_filtro 1]
  Fase_B : TransferFcn  Denominator=[1/(w_filtro)^2 2/w_filtro 1]
  Mux1 : Mux  Inputs=2
  Mux14 : Mux  Inputs=2
  Mux2 : Mux  Inputs=2
  Ia_mis_rete : Outport
  I_mis_scope : Outport  Port=2
  I_scope : Outport  Port=3
  wires:
  Fase_B/1 -> Mux1/2, Mux14/2
  Ia_rete/1 -> Mux2/1, Fase_A/1
  Mux2/1 -> I_scope/1
  Mux14/1 -> I_mis_scope/1
  Ib_rete/1 -> Fase_B/1, Mux2/2
  Mux1/1 -> Ia_mis_rete/1
  Fase_A/1 -> Mux1/1, Mux14/1

== system Filter_attivo/Inverter ==
  1 : Inport
  2 : Inport  Port=2
  " 1 " : DataTypeConversion  SaturateOnIntegerOverflow=on  RndMeth=Zero
  " 2 " : DataTypeConversion  SaturateOnIntegerOverflow=on  RndMeth=Zero
  " InputMux " : Mux  Inputs=2
  " S-Function " : S-Function  FunctionName=plecs  SFunctionDeploymentMode=off  EnableBusSupport=off
  wires:
  " InputMux "/1 -> " S-Function "/1
  1/1 -> " 1 "/1
  " 1 "/1 -> " InputMux "/1
  2/1 -> " 2 "/1
  " 2 "/1 -> " InputMux "/2

== system Filter_attivo/Inverter  ==
  va* : Inport
  vb* : Inport  Port=2
  vc* : Inport  Port=3
  In4 : Inport  Port=4
  C : powerlib/Elements/Series RLC Branch  LConnTagsString=__new0  RConnTagsString=__new0  BranchType=C  Resistance=1  Inductance=1e-3  SetiL0=off  InitialCurrent=0  Capacitance=C  Setx0=on  InitialVoltage=V_cond_iniz  Measurements=None
  Inverter trifase : Subsystem
  Modulatore PWM Simmetrica : Subsystem
  R : powerlib/Elements/Series RLC Branch  LConnTagsString=__new0  RConnTagsString=__new0  BranchType=R  Resistance=R_carico  Inductance=1e-3  SetiL0=off  InitialCurrent=0  Capacitance=1e-6  Setx0=off  InitialVoltage=0  Measurements=None
  Scope_idc : Subsystem  LoadFcn=plecs('sl', 300);  InitFcn=plecs('sl', 314);  StartFcn=plecs('sl', 308);  StopFcn=plecs('sl', 309);  mask{Settings=<binary blob, 876 chars, not shown>}
      mask init:
      | plecs('sl', 315);
      settings: CopyFcn=plecs('sl', 303);  DeleteFcn=plecs('sl', 305);  UndoDeleteFcn=plecs('sl', 306);  PreSaveFcn=plecs('sl', 311);  NameChangeFcn=plecs('sl', 310);  DestroyFcn=plecs('sl', 307);  OpenFcn=plecs('sl', 302);  ErrorFcn=plerrorfcn
      mask Display: plot([0.1 0.9 0.9 0.1 0.1], [0.9 0.9 0.5 0.5 0.9])
  Scope_idc_media : Subsystem  LoadFcn=plecs('sl', 300);  InitFcn=plecs('sl', 314);  StartFcn=plecs('sl', 308);  StopFcn=plecs('sl', 309);  mask{Settings=<binary blob, 892 chars, not shown>}
      mask init:
      | plecs('sl', 315);
      settings: CopyFcn=plecs('sl', 303);  DeleteFcn=plecs('sl', 305);  UndoDeleteFcn=plecs('sl', 306);  PreSaveFcn=plecs('sl', 311);  NameChangeFcn=plecs('sl', 310);  DestroyFcn=plecs('sl', 307);  OpenFcn=plecs('sl', 302);  ErrorFcn=plerrorfcn
      mask Display: plot([0.1 0.9 0.9 0.1 0.1], [0.9 0.9 0.5 0.5 0.9])
  Valore medio corrente : powerlib_extras/Measurements/Mean Value  Period=T
  Vdc : powerlib/Measurements/Voltage Measurement  PhasorSimulation=off  OutputType=Complex  PSBequivalent=0
  idc : powerlib/Measurements/Current Measurement  PhasorSimulation=off  OutputType=Complex  PSBequivalent=0
  va_inv : PMIOPort  Port=1  Side=Right
  vb_inv : PMIOPort  Port=2  Side=Right
  vc_inv : PMIOPort  Port=3  Side=Right
  Bus DC : Outport
  wires:
  Modulatore PWM Simmetrica/3(sb+) -> Inverter trifase/3(sb+)
  idc/1 -> Valore medio corrente/1, Scope_idc/1(1)
  Modulatore PWM Simmetrica/6(sc-) -> Inverter trifase/6(sc-)
  Vdc/1 -> Bus DC/1, [Vdc]
  Modulatore PWM Simmetrica/2(sa-) -> Inverter trifase/2(sa-)
  vb*/1 -> Modulatore PWM Simmetrica/2(vBN_ref)
  va*/1 -> Modulatore PWM Simmetrica/1(vAN_ref)
  [Vdc] -> Modulatore PWM Simmetrica/4(Vdc)
  Valore medio corrente/1 -> Scope_idc_media/1(1)
  Modulatore PWM Simmetrica/4(sb-) -> Inverter trifase/4(sb-)
  Modulatore PWM Simmetrica/5(sc+) -> Inverter trifase/5(sc+)
  Modulatore PWM Simmetrica/1(sa+) -> Inverter trifase/1(sa+)
  vc*/1 -> Modulatore PWM Simmetrica/3(vCN_ref)
  In4/1 -> Inverter trifase/7(Protezione)
  connections:
  C/LConn1 -- idc/LConn1 -- Vdc/LConn1
  Vdc/LConn2 -- C/RConn1 -- Inverter trifase/LConn2
  vc_inv/RConn1 -- Inverter trifase/RConn3
  Inverter trifase/LConn1 -- idc/RConn1
  vb_inv/RConn1 -- Inverter trifase/RConn2
  va_inv/RConn1 -- Inverter trifase/RConn1

== system Filter_attivo/Inverter1 ==
  1 : Inport
  2 : Inport  Port=2
  " 1 " : DataTypeConversion  SaturateOnIntegerOverflow=on  RndMeth=Zero
  " 2 " : DataTypeConversion  SaturateOnIntegerOverflow=on  RndMeth=Zero
  " InputMux " : Mux  Inputs=2
  " S-Function " : S-Function  FunctionName=plecs  SFunctionDeploymentMode=off  EnableBusSupport=off
  wires:
  " 2 "/1 -> " InputMux "/2
  2/1 -> " 2 "/1
  " 1 "/1 -> " InputMux "/1
  1/1 -> " 1 "/1
  " InputMux "/1 -> " S-Function "/1

== system Filter_attivo/Protezione ==
  Vdc : Inport
  Avvio_inverter : Inport  Port=2
  Limite down : Constant  Value=limite_down
  Limite up1 : Constant  Value=limite_up
  Logical Operator : Logic  Inputs=3  AllPortsSameDT=off  OutDataTypeStr=boolean
  Relational Operator : RelationalOperator  OutDataTypeStr=boolean  RndMeth=Nearest
  Relational Operator1 : RelationalOperator  Operator=<=  OutDataTypeStr=boolean  RndMeth=Nearest
  Scope : Subsystem  LoadFcn=plecs('sl', 300);  InitFcn=plecs('sl', 314);  StartFcn=plecs('sl', 308);  StopFcn=plecs('sl', 309);  mask{Settings=<binary blob, 1148 chars, not shown>}
      mask init:
      | plecs('sl', 315);
      settings: CopyFcn=plecs('sl', 303);  DeleteFcn=plecs('sl', 305);  UndoDeleteFcn=plecs('sl', 306);  PreSaveFcn=plecs('sl', 311);  NameChangeFcn=plecs('sl', 310);  DestroyFcn=plecs('sl', 307);  OpenFcn=plecs('sl', 302);  ErrorFcn=plerrorfcn
      mask Display: plot([0.1 0.9 0.9 0.1 0.1], [0.9 0.9 0.5 0.5 0.9])
  "Protezione " : Outport
  wires:
  Logical Operator/1 -> "Protezione "/1
  Limite down/1 -> Relational Operator1/1
  Relational Operator1/1 -> Scope/2(2), Logical Operator/2
  Relational Operator/1 -> Scope/1(1), Logical Operator/1
  Vdc/1 -> Relational Operator1/2, Relational Operator/2
  Avvio_inverter/1 -> Scope/3(3), Logical Operator/3
  Limite up1/1 -> Relational Operator/1

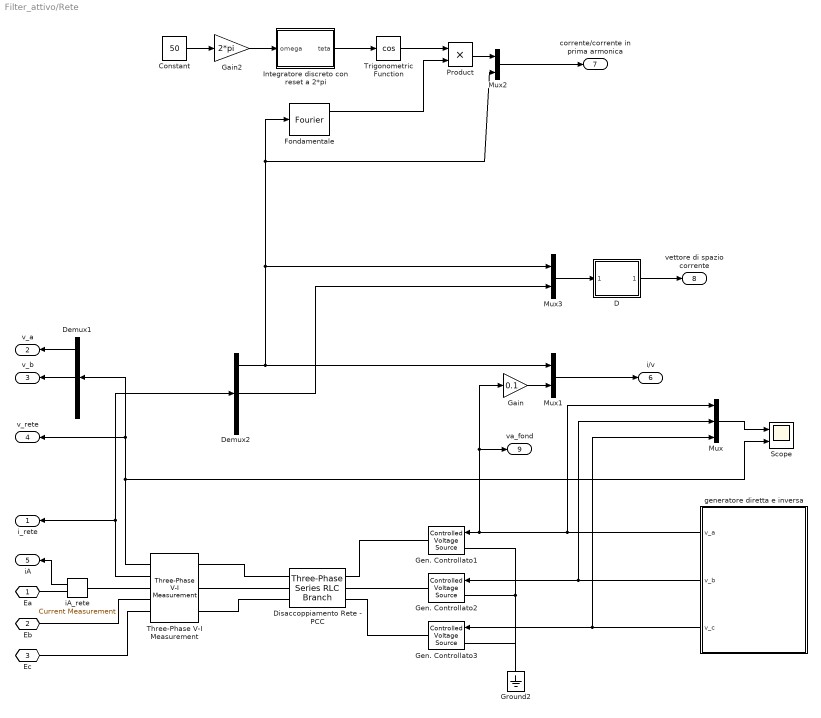
== system Filter_attivo/Rete ==
  Constant : Constant  Value=50
  D : Subsystem
  Demux1 : Demux  Outputs=3
  Demux2 : Demux  Outputs=3
  Disaccoppiamento Rete - PCC : powerlib/Elements/Three-Phase Series RLC Branch  LConnTagsString=A|B|C  RConnTagsString=A|B|C  BranchType=RL  Resistance=R_rete  Inductance=L_rete  Capacitance=1e-6  Measurements=Branch currents
  Fondamentale : powerlib_meascontrol/Measurements/Fourier  Freq=50  n=1  InInit=[0, 0]  Ts=0
  Gain : Gain  Gain=0.1
  Gain2 : Gain  Gain=2*pi
  Gen. Controllato1 : powerlib/Electrical Sources/Controlled Voltage Source  Initialize=on  Source_Type=AC  Amplitude=0  Phase=0  Frequency=0  Measurements=None
  Gen. Controllato2 : powerlib/Electrical Sources/Controlled Voltage Source  Initialize=on  Source_Type=AC  Amplitude=0  Phase=0  Frequency=0  Measurements=None
  Gen. Controllato3 : powerlib/Electrical Sources/Controlled Voltage Source  Initialize=on  Source_Type=AC  Amplitude=0  Phase=0  Frequency=0  Measurements=None
  Ground2 : powerlib/Elements/Ground  LConnTagsString=a
  Integratore discreto con reset a 2*pi : Subsystem
  Mux : Mux  Inputs=3
  Mux1 : Mux  Inputs=2
  Mux2 : Mux  Inputs=2
  Mux3 : Mux  Inputs=2
  Product : Product
  Scope : Scope  NumInputPorts=2
  Three-Phase V-I Measurement : powerlib/Measurements/Three-Phase V-I Measurement  VoltageMeasurement=phase-to-ground  SetLabelV=off  LabelV=Vabc  Vpu=off  VpuLL=off  CurrentMeasurement=yes  SetLabelI=off  LabelI=Iabc  Ipu=off  Pbase=100e6  Vbase=500e3  OutputType=Complex  PhasorSimulation=off  PSBequivalent=0
  Trigonometric Function : Trigonometry  Operator=cos
  generatore diretta e inversa : Subsystem  mask{fase_i=12.5, ampiezza_i=0}
      mask prompts: fase_i "fase inversa in gradi"; ampiezza_i "ampiezza inversa P.U."
  iA_rete : powerlib/Measurements/Current Measurement  PhasorSimulation=off  OutputType=Complex  PSBequivalent=0
  Ea : PMIOPort  Port=1  Side=Left
  Eb : PMIOPort  Port=2  Side=Left
  Ec : PMIOPort  Port=3  Side=Left
  "i_rete " : Outport
  v_a : Outport  Port=2
  v_b : Outport  Port=3
  "v_rete " : Outport  Port=4
  iA : Outport  Port=5
  i/v : Outport  Port=6
  corrente/corrente in prima armonica : Outport  Port=7
  vettore di spazio corrente : Outport  Port=8
  va_fond : Outport  Port=9
  wires:
  Three-Phase V-I Measurement/1 -> Scope/2, Demux1/1, "v_rete "/1
  Three-Phase V-I Measurement/2 -> Demux2/1, "i_rete "/1
  Demux1/1 -> v_a/1
  Demux1/2 -> v_b/1
  iA_rete/1 -> iA/1
  generatore diretta e inversa/1(v_a) -> Mux/1, va_fond/1, Gain/1, Gen. Controllato1/1
  generatore diretta e inversa/2(v_b) -> Mux/2, Gen. Controllato2/1
  generatore diretta e inversa/3(v_c) -> Mux/3, Gen. Controllato3/1
  Mux1/1 -> i/v/1
  Demux2/1 -> Mux3/1, Mux2/2, Fondamentale/1, Mux1/1
  Gain/1 -> Mux1/2
  Gain2/1 -> Integratore discreto con reset a 2*pi/1(omega)
  Constant/1 -> Gain2/1
  Integratore discreto con reset a 2*pi/1(teta) -> Trigonometric Function/1
  Trigonometric Function/1 -> Product/1
  Fondamentale/1 -> Product/2
  Product/1 -> Mux2/1
  Mux2/1 -> corrente/corrente in prima armonica/1
  Demux2/2 -> Mux3/2
  Mux3/1 -> D/1(ab(c))
  D/1(dq(0)) -> vettore di spazio corrente/1
  Mux/1 -> Scope/1
  connections:
  iA_rete/RConn1 -- Ea/RConn1
  Ground2/LConn1 -- Gen. Controllato3/LConn1 -- Gen. Controllato1/LConn1 -- Gen. Controllato2/LConn1
  Three-Phase V-I Measurement/RConn1 -- iA_rete/LConn1
  Three-Phase V-I Measurement/RConn2 -- Eb/RConn1
  Three-Phase V-I Measurement/RConn3 -- Ec/RConn1
  Disaccoppiamento Rete - PCC/LConn2 -- Three-Phase V-I Measurement/LConn2
  Disaccoppiamento Rete - PCC/RConn2 -- Gen. Controllato2/RConn1
  Gen. Controllato1/RConn1 -- Disaccoppiamento Rete - PCC/RConn1
  Gen. Controllato3/RConn1 -- Disaccoppiamento Rete - PCC/RConn3
  Disaccoppiamento Rete - PCC/LConn3 -- Three-Phase V-I Measurement/LConn3
  Three-Phase V-I Measurement/LConn1 -- Disaccoppiamento Rete - PCC/LConn1

== system Filter_attivo/Scope ==
  1 : Inport
  2 : Inport  Port=2
  3 : Inport  Port=3
  " 1 " : DataTypeConversion  SaturateOnIntegerOverflow=on  RndMeth=Zero
  " 2 " : DataTypeConversion  SaturateOnIntegerOverflow=on  RndMeth=Zero
  " 3 " : DataTypeConversion  SaturateOnIntegerOverflow=on  RndMeth=Zero
  " InputMux " : Mux  Inputs=3
  " S-Function " : S-Function  FunctionName=plecs  SFunctionDeploymentMode=off  EnableBusSupport=off
  wires:
  " InputMux "/1 -> " S-Function "/1
  1/1 -> " 1 "/1
  " 1 "/1 -> " InputMux "/1
  2/1 -> " 2 "/1
  " 2 "/1 -> " InputMux "/2
  3/1 -> " 3 "/1
  " 3 "/1 -> " InputMux "/3

== system Filter_attivo/Scope1 ==
  1 : Inport
  " InputMux " : Subsystem
      mask Display: disp('Mux')
  " S-Function " : S-Function  FunctionName=plecs  SFunctionDeploymentMode=off  EnableBusSupport=off
  wires:
  1/1 -> " InputMux "/1(In1)
  " InputMux "/1(Out) -> " S-Function "/1

== system Filter_attivo/Scope2 ==
  1 : Inport
  " InputMux " : Subsystem
      mask Display: disp('Mux')
  " S-Function " : S-Function  FunctionName=plecs  SFunctionDeploymentMode=off  EnableBusSupport=off
  wires:
  " InputMux "/1(Out) -> " S-Function "/1
  1/1 -> " InputMux "/1(In1)

== system Filter_attivo/Scope3 ==
  1 : Inport
  " 1 " : DataTypeConversion  SaturateOnIntegerOverflow=on  RndMeth=Zero
  " InputMux " : Mux  Inputs=1
  " S-Function " : S-Function  FunctionName=plecs  SFunctionDeploymentMode=off  EnableBusSupport=off
  wires:
  " InputMux "/1 -> " S-Function "/1
  1/1 -> " 1 "/1
  " 1 "/1 -> " InputMux "/1

== system Filter_attivo/Subsystem ==
  Ground1 : powerlib/Elements/Ground  LConnTagsString=a
  Ground2 : powerlib/Elements/Ground  LConnTagsString=a
  Imedenza disaccoppiamento Carico - PCC1 : powerlib/Elements/Three-Phase Series RLC Branch  LConnTagsString=A|B|C  RConnTagsString=A|B|C  BranchType=RL  Resistance=R_disaccoppiamento  Inductance=0.13/4  Capacitance=1e-6  Measurements=None
  Series RLC Branch : powerlib/Elements/Series RLC Branch  LConnTagsString=__new0  RConnTagsString=__new0  BranchType=R  Resistance=50  Inductance=1e-3  SetiL0=off  InitialCurrent=0  Capacitance=1e-6  Setx0=off  InitialVoltage=0  Measurements=None
  Conn1 : PMIOPort  Port=1  Side=Right
  Conn2 : PMIOPort  Port=2  Side=Right
  "Conn3 " : PMIOPort  Port=3  Side=Right
  connections:
  Imedenza disaccoppiamento Carico - PCC1/RConn2 -- Conn2/RConn1
  Imedenza disaccoppiamento Carico - PCC1/RConn3 -- "Conn3 "/RConn1
  Imedenza disaccoppiamento Carico - PCC1/RConn1 -- Series RLC Branch/LConn1 -- Conn1/RConn1
  Ground2/LConn1 -- Imedenza disaccoppiamento Carico - PCC1/LConn1 -- Imedenza disaccoppiamento Carico - PCC1/LConn3 -- Imedenza disaccoppiamento Carico - PCC1/LConn2
  Ground1/LConn1 -- Series RLC Branch/RConn1

== system Filter_attivo/Tensione bus DC ==
  1 : Inport
  " InputMux " : Subsystem
      mask Display: disp('Mux')
  " S-Function " : S-Function  FunctionName=plecs  SFunctionDeploymentMode=off  EnableBusSupport=off
  wires:
  1/1 -> " InputMux "/1(In1)
  " InputMux "/1(Out) -> " S-Function "/1

== system Filter_attivo/Vconcatenate a Vfase inverter ==
  V12 : Inport
  V23 : Inport  Port=2
  V31 : Inport  Port=3
  Add{,1..5} (6 alike) : Sum  Inputs=+-
  Add6 : Sum  Inputs=+++
  Gain{,1..3} (4 alike) : Gain  Gain=1/3
  E1 : Outport
  E2 : Outport  Port=2
  E3 : Outport  Port=3
  wires:
  V12/1 -> Add/1, Add1/2
  V23/1 -> Add1/1, Add2/2
  V31/1 -> Add2/1, Add/2
  Add/1 -> Gain/1
  Add1/1 -> Gain1/1
  Add2/1 -> Gain2/1
  Gain/1 -> Add3/1, Add6/1
  Gain1/1 -> Add4/1, Add6/2
  Gain2/1 -> Add5/1, Add6/3
  Add6/1 -> Gain3/1
  Gain3/1 -> Add3/2, Add4/2, Add5/2
  Add3/1 -> E1/1
  Add4/1 -> E2/1
  Add5/1 -> E3/1

== system Filter_attivo/XY Plot ==
  1 : Inport
  2 : Inport  Port=2
  " InputMux " : Subsystem
      mask Display: disp('Mux')
  " S-Function " : S-Function  FunctionName=plecs  SFunctionDeploymentMode=off  EnableBusSupport=off
  wires:
  2/1 -> " InputMux "/1(In1)
  1/1 -> " InputMux "/2(In2)
  " InputMux "/1(Out) -> " S-Function "/1

== system Filter_attivo/iA_media ==
  1 : Inport
  " 1 " : DataTypeConversion  SaturateOnIntegerOverflow=on  RndMeth=Zero
  " InputMux " : Mux  Inputs=1
  " S-Function " : S-Function  FunctionName=plecs  SFunctionDeploymentMode=off  EnableBusSupport=off
  wires:
  " 1 "/1 -> " InputMux "/1
  1/1 -> " 1 "/1
  " InputMux "/1 -> " S-Function "/1

== system Filter_attivo/i_rete ==
  1 : Inport
  " 1 " : DataTypeConversion  SaturateOnIntegerOverflow=on  RndMeth=Zero
  " InputMux " : Mux  Inputs=1
  " S-Function " : S-Function  FunctionName=plecs  SFunctionDeploymentMode=off  EnableBusSupport=off
  wires:
  " InputMux "/1 -> " S-Function "/1
  1/1 -> " 1 "/1
  " 1 "/1 -> " InputMux "/1

== system Filter_attivo/v_rete ==
  1 : Inport
  " InputMux " : Subsystem
      mask Display: disp('Mux')
  " S-Function " : S-Function  FunctionName=plecs  SFunctionDeploymentMode=off  EnableBusSupport=off
  wires:
  " InputMux "/1(Out) -> " S-Function "/1
  1/1 -> " InputMux "/1(In1)

== system Filter_attivo/v_rete1 ==
  1 : Inport
  " InputMux " : Subsystem
      mask Display: disp('Mux')
  " S-Function " : S-Function  FunctionName=plecs  SFunctionDeploymentMode=off  EnableBusSupport=off
  wires:
  1/1 -> " InputMux "/1(In1)
  " InputMux "/1(Out) -> " S-Function "/1

== system Filter_attivo/Carico non lineare/Ponte raddrizzatore ==
  DA+ : powerlib/Power Electronics/Diode  Ron=0.001  Lon=0  Vf=0.8  IC=0  UseSnubber=off  Rs=500  Cs=250e-9  Measurements=off
  DA- : powerlib/Power Electronics/Diode  Ron=0.001  Lon=0  Vf=0.8  IC=0  UseSnubber=off  Rs=500  Cs=250e-9  Measurements=off
  DB+ : powerlib/Power Electronics/Diode  Ron=0.001  Lon=0  Vf=0.8  IC=0  UseSnubber=off  Rs=500  Cs=250e-9  Measurements=off
  DB- : powerlib/Power Electronics/Diode  Ron=0.001  Lon=0  Vf=0.8  IC=0  UseSnubber=off  Rs=500  Cs=250e-9  Measurements=off
  DC+ : powerlib/Power Electronics/Diode  Ron=0.001  Lon=0  Vf=0.8  IC=0  UseSnubber=off  Rs=500  Cs=250e-9  Measurements=off
  DC- : powerlib/Power Electronics/Diode  Ron=0.001  Lon=0  Vf=0.8  IC=0  UseSnubber=off  Rs=500  Cs=250e-9  Measurements=off
  A : PMIOPort  Tag=PMCPort  Port=1  Side=Left
  B : PMIOPort  Tag=PMCPort  Port=2  Side=Left
  C : PMIOPort  Tag=PMCPort  Port=3  Side=Left
  v+ : PMIOPort  Tag=PMCPort  Port=4  Side=Right
  v- : PMIOPort  Tag=PMCPort  Port=5  Side=Right
  connections:
  DB-/LConn1 -- v-/RConn1 -- DC-/LConn1 -- DA-/LConn1
  DA+/LConn1 -- A/RConn1 -- DA-/RConn1
  DB+/RConn1 -- v+/RConn1 -- DC+/RConn1 -- DA+/RConn1
  DB-/RConn1 -- B/RConn1 -- DB+/LConn1
  DC+/LConn1 -- C/RConn1 -- DC-/RConn1

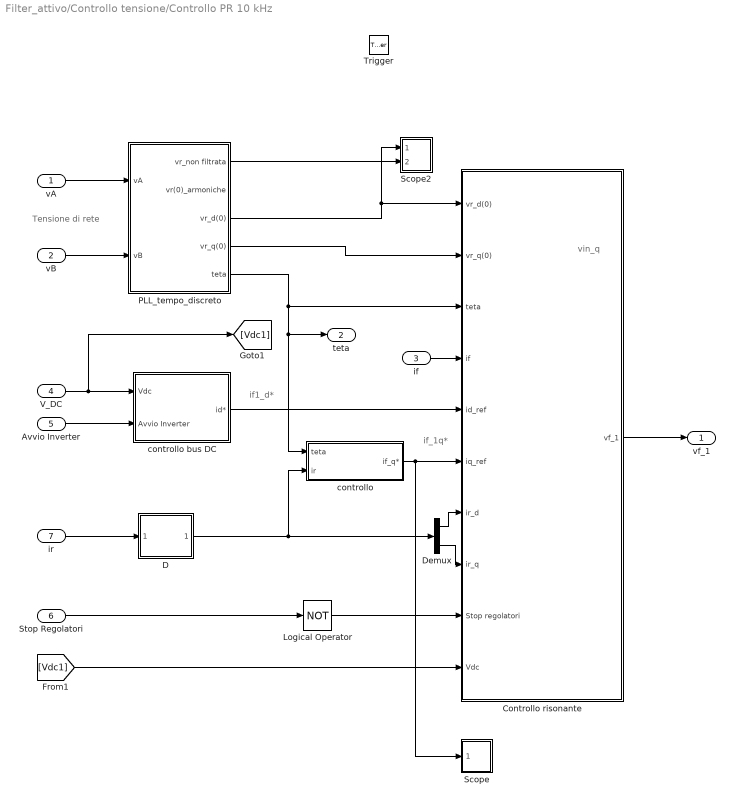
== system Filter_attivo/Controllo tensione/Controllo PR 10 kHz ==
  note: Tensione di rete
  note: if1_d*
  note: vin_q
  note: if_1q*
  vA : Inport
  vB : Inport  Port=2
  if : Inport  Port=3
  V_DC : Inport  Port=4
  Avvio Inverter : Inport  Port=5
  Stop Regolatori : Inport  Port=6
  ir : Inport  Port=7
  Trigger : TriggerPort  VariantControl=Variant
  Controllo risonante : Subsystem
  D : Subsystem
  Demux : Demux  Outputs=2
  Logical Operator : Logic  Operator=NOT  AllPortsSameDT=off  OutDataTypeStr=boolean
  PLL_tempo_discreto : Subsystem
  Scope : Subsystem  LoadFcn=plecs('sl', 300);  InitFcn=plecs('sl', 314);  StartFcn=plecs('sl', 308);  StopFcn=plecs('sl', 309);  mask{Settings=<binary blob, 892 chars, not shown>}
      mask init:
      | plecs('sl', 315);
      settings: CopyFcn=plecs('sl', 303);  DeleteFcn=plecs('sl', 305);  UndoDeleteFcn=plecs('sl', 306);  PreSaveFcn=plecs('sl', 311);  NameChangeFcn=plecs('sl', 310);  DestroyFcn=plecs('sl', 307);  OpenFcn=plecs('sl', 302);  ErrorFcn=plerrorfcn
      mask Display: plot([0.1 0.9 0.9 0.1 0.1], [0.9 0.9 0.5 0.5 0.9])
  Scope2 : Subsystem  LoadFcn=plecs('sl', 300);  InitFcn=plecs('sl', 314);  StartFcn=plecs('sl', 308);  StopFcn=plecs('sl', 309);  mask{Settings=<binary blob, 1020 chars, not shown>}
      mask init:
      | plecs('sl', 315);
      settings: CopyFcn=plecs('sl', 303);  DeleteFcn=plecs('sl', 305);  UndoDeleteFcn=plecs('sl', 306);  PreSaveFcn=plecs('sl', 311);  NameChangeFcn=plecs('sl', 310);  DestroyFcn=plecs('sl', 307);  OpenFcn=plecs('sl', 302);  ErrorFcn=plerrorfcn
      mask Display: plot([0.1 0.9 0.9 0.1 0.1], [0.9 0.9 0.5 0.5 0.9])
  "controllo " : Subsystem  mask{avvio_rifasamento=0.4}
      mask prompts: avvio_rifasamento "avvio controllo rifasamento"
  controllo bus DC : Subsystem
  vf_1 : Outport
  teta : Outport  Port=2
  wires:
  D/1(dq(0)) -> "controllo "/2(ir), Demux/1
  Stop Regolatori/1 -> Logical Operator/1
  Demux/2 -> Controllo risonante/8(ir_q)
  ir/1 -> D/1(ab(c))
  PLL_tempo_discreto/4(vr_q(0)) -> Controllo risonante/2(vr_q(0))
  PLL_tempo_discreto/3(vr_d(0)) -> Scope2/1(1), Controllo risonante/1(vr_d(0))
  if/1 -> Controllo risonante/4(if)
  Demux/1 -> Controllo risonante/7(ir_d)
  vA/1 -> PLL_tempo_discreto/1(vA)
  vB/1 -> PLL_tempo_discreto/2(vB)
  Logical Operator/1 -> Controllo risonante/9(Stop regolatori)
  PLL_tempo_discreto/1(vr_non filtrata) -> Scope2/2(2)
  PLL_tempo_discreto/5(teta) -> teta/1, "controllo "/1(teta), Controllo risonante/3(teta)
  controllo bus DC/1(id*) -> Controllo risonante/5(id_ref)
  "controllo "/1(if_q*) -> Scope/1(1), Controllo risonante/6(iq_ref)
  Avvio Inverter/1 -> controllo bus DC/2(Avvio Inverter)
  [Vdc1] -> Controllo risonante/10(Vdc)
  V_DC/1 -> controllo bus DC/1(Vdc), [Vdc1]
  Controllo risonante/1(vf_1) -> vf_1/1

== system Filter_attivo/Controllo tensione/Controllo ripetitivo ==
  protezione : Inport
  ir : Inport  Port=2
  teta : Inport  Port=3
  Constant : Constant  Value=alfa
  Controllo ripetitivo : Subsystem
  Controllo ripetitivo con downsampling : Subsystem
  Generatore a fc : DiscretePulseGenerator  PulseType=Time based  Period=Tc
  Generatore a frequenza variabile : DiscretePulseGenerator  PulseType=Time based  Period=down*Tc
  Notch Prima Armonica : Subsystem
  Step1 : Step  Time=time_to_rip  SampleTime=0
  Switch : Switch  Criteria=u2 > Threshold
  vf_h : Outport
  wires:
  Generatore a frequenza variabile/1 -> Controllo ripetitivo con downsampling/Trigger
  protezione/1 -> Controllo ripetitivo/1(Stop regolatori), Controllo ripetitivo con downsampling/1(Stop regolatori)
  Step1/1 -> Controllo ripetitivo/2(Avvio ripetitivo), Controllo ripetitivo con downsampling/2(Avvio ripetitivo)
  teta/1 -> Controllo ripetitivo/4(teta)
  Generatore a fc/1 -> [clock_10kHz]
  [clock_10kHz] -> Notch Prima Armonica/Trigger
  [clock_10kHz] -> Controllo ripetitivo/Trigger
  Controllo ripetitivo con downsampling/1(vf_h_DOWNSAMPLING) -> Switch/1
  Switch/1 -> vf_h/1
  Controllo ripetitivo/1(vf_h) -> Switch/3
  Constant/1 -> Switch/2
  ir/1 -> Notch Prima Armonica/1(ir(a_b_c))
  Notch Prima Armonica/1(ir_h(d_q)) -> Controllo ripetitivo/3("corrente rete "), Controllo ripetitivo con downsampling/3("corrente rete ")

== system Filter_attivo/Controllo tensione/Scope ==
  1 : Inport
  " InputMux " : Subsystem
      mask Display: disp('Mux')
  " S-Function " : S-Function  FunctionName=plecs  SFunctionDeploymentMode=off  EnableBusSupport=off
  wires:
  1/1 -> " InputMux "/1(In1)
  " InputMux "/1(Out) -> " S-Function "/1

== system Filter_attivo/Controllo tensione/Scope1 ==
  1 : Inport
  2 : Inport  Port=2
  " 1 " : DataTypeConversion  SaturateOnIntegerOverflow=on  RndMeth=Zero
  " 2 " : DataTypeConversion  SaturateOnIntegerOverflow=on  RndMeth=Zero
  " InputMux " : Mux  Inputs=2
  " S-Function " : S-Function  FunctionName=plecs  SFunctionDeploymentMode=off  EnableBusSupport=off
  wires:
  " InputMux "/1 -> " S-Function "/1
  1/1 -> " 1 "/1
  " 1 "/1 -> " InputMux "/1
  2/1 -> " 2 "/1
  " 2 "/1 -> " InputMux "/2

== system Filter_attivo/Controllo tensione/Scope2 ==
  1 : Inport
  " InputMux " : Subsystem
      mask Display: disp('Mux')
  " S-Function " : S-Function  FunctionName=plecs  SFunctionDeploymentMode=off  EnableBusSupport=off
  wires:
  1/1 -> " InputMux "/1(In1)
  " InputMux "/1(Out) -> " S-Function "/1

== system Filter_attivo/Controllo tensione/inv_D ==
  dq(0) : Inport
  Gain : Gain  Gain=[1 0; -1/2 sqrt(3)/2]  Multiplication=Matrix(K*u)
  ab(c) : Outport
  wires:
  Gain/1 -> ab(c)/1
  dq(0)/1 -> Gain/1

== system Filter_attivo/Filtro di sallen Key correnti inverter /D ==
  ab(c) : Inport
  Gain : Gain  Gain=[1 0; 1/sqrt(3) 2/sqrt(3)]  Multiplication=Matrix(K*u)
  dq(0) : Outport
  wires:
  Gain/1 -> dq(0)/1
  ab(c)/1 -> Gain/1
